simulink model "Q2"  (R2015b)
settings: Solver=FixedStepAuto  StartTime=0.0  StopTime=1  FixedStep=0.002  RelTol=1e-3
values from neighbouring files (symbols this model uses):
  J = 5    [Q1e.m]    (also in Q1i.m; Q2biv.m = 4.32e-07)
  K = 0.05    [Q1e.m]    (also in Q1i.m = 167.9832; Q2biv.m = 0.0119)
  K_d = 39.3    [Q1i.m]    (also in Q2biv.m = 0.000305)
  PID_K_d = K    (= 0.0119)    [Q2biv.m]
  PID_K_i = (Z*I)*PID_K_d    [Q2biv.m]
  PID_K_p = (Z+I)*PID_K_d    [Q2biv.m]
settings Model: Creator=SooJengTan  LastModifiedBy=SooJengTan

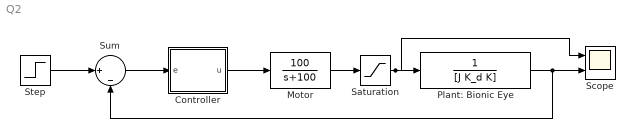
== system Q2 ==
  Controller : Subsystem
  Motor : TransferFcn  Numerator=[100]  Denominator=[1 100]
  Plant: Bionic Eye : TransferFcn  Denominator=[J K_d K]
  Saturation : Saturate
  Scope : Scope  NumInputPorts=2
  Step : Step  Time=0  SampleTime=0
  Sum : Sum  Inputs=||+|-
  wires:
  Step/1 -> Sum/1
  Sum/1 -> Controller/1(e)
  Motor/1 -> Saturation/1
  Saturation/1 -> Scope/1, Plant: Bionic Eye/1
  Controller/1(u) -> Motor/1
  Plant: Bionic Eye/1 -> Sum/2, Scope/2

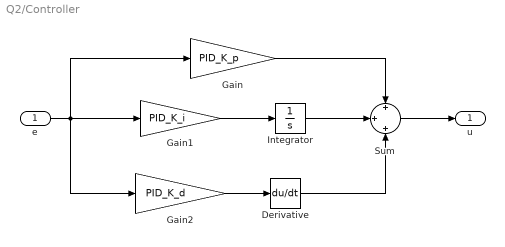
== system Q2/Controller ==
  e : Inport
  Derivative : Derivative
  Gain : Gain  Gain=PID_K_p
  Gain1 : Gain  Gain=PID_K_i
  Gain2 : Gain  Gain=PID_K_d
  Integrator : Integrator
  Sum : Sum  Inputs=+|+|+
  u : Outport
  wires:
  e/1 -> Gain2/1, Gain1/1, Gain/1
  Gain2/1 -> Derivative/1
  Gain1/1 -> Integrator/1
  Gain/1 -> Sum/1
  Derivative/1 -> Sum/3
  Integrator/1 -> Sum/2
  Sum/1 -> u/1
